simulink model "TParkDir"  (R2020b)
settings: Solver=VariableStepAuto  StartTime=0.0  StopTime=10.0  RelTol=1e-3
values from neighbouring files (symbols this model uses):
  beq = bm+(blnom/(r^2))    (= 1.5e-05)    [valores.m]
  Jeq = (Jm+Jl/r^2)    (= 5.65099476805e-06)    [Valores_de_Parametros.m]    (also in valores.m)
  lambda_m = 0.01546    [Valores_de_Parametros.m]    (also in valores.m)
  Ld = 6.6    [Valores_de_Parametros.m]    (also in valores.m = 0.0066)
  Lls = 0.8    [Valores_de_Parametros.m]    (also in valores.m = 0.0008)
  Lq = 5.8    [Valores_de_Parametros.m]    (also in valores.m = 0.0058)
  Pp = 3    [Valores_de_Parametros.m]    (also in valores.m)
  r = 314.3008    [Valores_de_Parametros.m]    (also in valores.m)
  Rs = 1.02    [Valores_de_Parametros.m]    (also in valores.m)
settings Model: Creator=Matias  LastModifiedBy=Matias

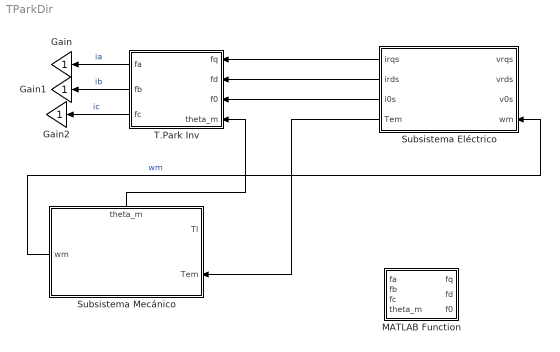
== system TParkDir ==
  Gain : Gain
  Gain1 : Gain
  Gain2 : Gain
  MATLAB Function : MATLAB Function  TreatAsAtomicUnit=on
  Subsistema Eléctrico : Subsystem
  Subsistema Mecánico : Subsystem
      settings: PortSchema="{\"entries\":[{\"content\":{\"sides\":[{\"content\":{\"connectorIds\":[\"In1\",\"In2\"]},\"type\":\"ConnectorPlacement.EquallySpacedRectSide\",\"uuid\":\"ee0e19e9-1195-452b-ab3d-8be3dd040414\"},{\"content\":{\"connectorIds\":[\"Out1\"],\"side\":\"RIGHT\"},\"type\":\"ConnectorPlacement.EquallySpacedRectSide\",\"uuid\":\"524e54e6-4967-4b42-ae12-58774e9397a0\"},{\"content\":{\"connectorIds\":[\"Out2\"],\"side\":\"TOP\"},\"type\":\"ConnectorPlacement.EquallySpacedRectSide\",\"uuid\":\"fab71378-68cb-4446-b02c-df48705d1789\"},{\"content\":{\"connectorIds\":[],\"side\":\"HIDDEN\"},\"type\":\"ConnectorPlacement.EquallySpacedRectSide\",\"uuid\":\"eea92cb8-3517-43ef-96fe-10b46f054d59\"}]},\"type\":\"ConnectorPlacement.EquallySpacedConnector\",\"uuid\":\"156d3ac5-e5c7-4248-8590-4f82c7370a76\"}],\"packageUris\":[\"http://schema.mathworks.com/mf0/Connector/R2020b\"],\"version\":\"1.0\"}"
  T.Park Inv : MATLAB Function  TreatAsAtomicUnit=on
  wires:
  Subsistema Mecánico/1(wm) -> Subsistema Eléctrico/4(wm)  "wm"
  Subsistema Eléctrico/4(Tem) -> Subsistema Mecánico/2(Tem)
  Subsistema Eléctrico/1(irqs) -> T.Park Inv/1(fq)
  Subsistema Eléctrico/2(irds) -> T.Park Inv/2(fd)
  Subsistema Eléctrico/3(i0s) -> T.Park Inv/3(f0)
  Subsistema Mecánico/2(theta_m) -> T.Park Inv/4(theta_m)
  T.Park Inv/1(fa) -> Gain/1  "ia"
  T.Park Inv/2(fb) -> Gain1/1  "ib"
  T.Park Inv/3(fc) -> Gain2/1  "ic"

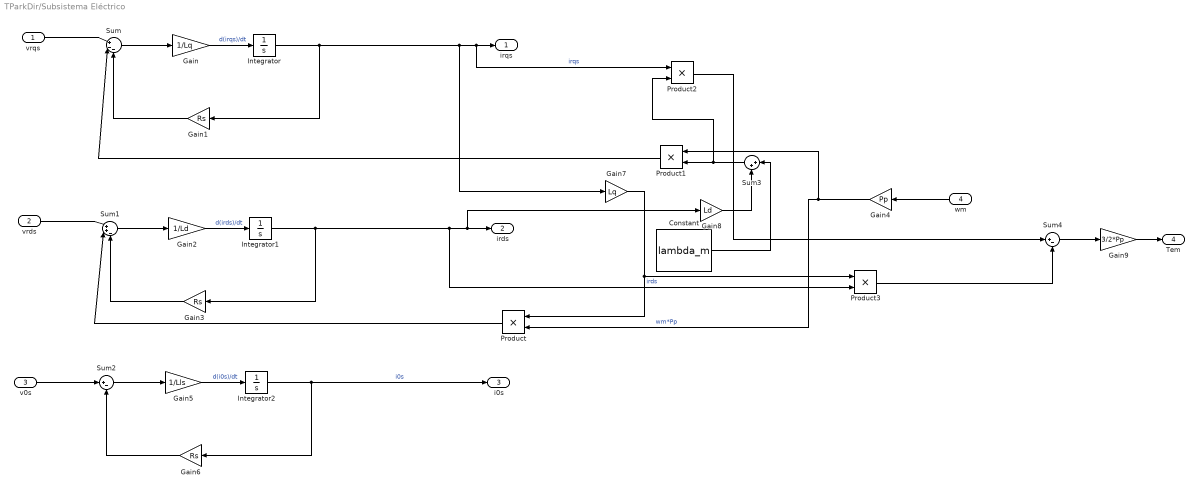
== system TParkDir/Subsistema Eléctrico ==
  vrqs : Inport
  vrds : Inport  Port=2
  v0s : Inport  Port=3
  wm : Inport  Port=4
  Constant : Constant  Value=lambda_m
  Gain : Gain  Gain=1/Lq
  Gain1 : Gain  Gain=Rs
  Gain2 : Gain  Gain=1/Ld
  Gain3 : Gain  Gain=Rs
  Gain4 : Gain  Gain=Pp
  Gain5 : Gain  Gain=1/Lls
  Gain6 : Gain  Gain=Rs
  Gain7 : Gain  Gain=Lq
  Gain8 : Gain  Gain=Ld
  Gain9 : Gain  Gain=3/2*Pp
  Integrator : Integrator
  Integrator1 : Integrator
  Integrator2 : Integrator
  Product{,1..3} (4 alike) : Product
  Sum : Sum  Inputs=|+--
  Sum1 : Sum  Inputs=|++-
  Sum2 : Sum  Inputs=|+-
  Sum3 : Sum  Inputs=|++
  Sum4 : Sum  Inputs=|+-
  irqs : Outport
  irds : Outport  Port=2
  i0s : Outport  Port=3
  Tem : Outport  Port=4
  wires:
  Sum3/1 -> Product2/2, Product1/2
  Integrator1/1 -> Gain3/1, Product3/2, Gain8/1, irds/1  "irds"
  Sum1/1 -> Gain2/1
  Gain8/1 -> Sum3/2
  Gain2/1 -> Integrator1/1  "d(irds)/dt"
  Product2/1 -> Sum4/1
  Constant/1 -> Sum3/1
  Gain3/1 -> Sum1/3
  Sum4/1 -> Gain9/1
  Product3/1 -> Sum4/2
  vrqs/1 -> Sum/1
  wm/1 -> Gain4/1
  vrds/1 -> Sum1/1
  Product/1 -> Sum1/2
  Product1/1 -> Sum/2
  v0s/1 -> Sum2/1
  Gain5/1 -> Integrator2/1  "d(i0s)/dt"
  Sum2/1 -> Gain5/1
  Integrator2/1 -> Gain6/1, i0s/1  "i0s"
  Gain4/1 -> Product1/1, Product/2  "wm*Pp"
  Sum/1 -> Gain/1
  Gain1/1 -> Sum/3
  Gain7/1 -> Product/1, Product3/1
  Integrator/1 -> Gain1/1, Gain7/1, Product2/1, irqs/1  "irqs"
  Gain/1 -> Integrator/1  "d(irqs)/dt"
  Gain9/1 -> Tem/1
  Gain6/1 -> Sum2/2

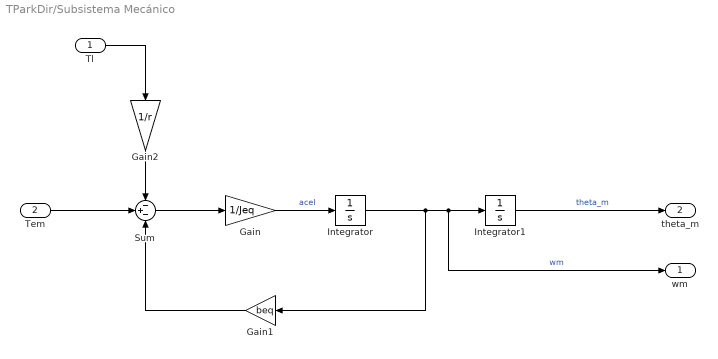
== system TParkDir/Subsistema Mecánico ==
  Tl : Inport
  Tem : Inport  Port=2
  Gain : Gain  Gain=1/Jeq
  Gain1 : Gain  Gain=beq
  Gain2 : Gain  Gain=1/r
  Integrator : Integrator
  Integrator1 : Integrator
  Sum : Sum  Inputs=-+-
  wm : Outport
  theta_m : Outport  Port=2
  wires:
  Sum/1 -> Gain/1
  Tl/1 -> Gain2/1
  Gain1/1 -> Sum/3
  Integrator/1 -> Gain1/1, wm/1, Integrator1/1  "wm"
  Gain2/1 -> Sum/1
  Gain/1 -> Integrator/1  "acel"
  Integrator1/1 -> theta_m/1  "theta_m"
  Tem/1 -> Sum/2

== matlab function TParkDir/MATLAB Function ==
  data: fa input; fq output; fb input; fc input; theta_m input; fd output; f0 output
function [fq,fd,f0] = fcn(fa,fb,fc,theta_m)
fq=2/3*(cos(theta_m)*fa+cos(theta_m-(2*pi/(3)))*fb+cos(theta_m+(2*pi/(3)))*fc);
fd=2/3*(sin(theta_m)*fa+sin(theta_m-(2*pi/(3)))*fb+sin(theta_m+(2*pi/(3)))*fc);
f0=2/3*((1/2)*fa+(1/2)*fb+(1/2)*fc);
y = u;

== matlab function TParkDir/T.Park Inv ==
  data: fq input; fa output; fd input; f0 input; theta_m input; fb output; fc output
function [fa,fb,fc] = fcn(fq,fd,f0,theta_m)
fa=fq*cos(theta_m)+fd*sin(theta_m)+f0;
fb=fq*cos(theta_m-(2*pi/(3)))+fd*sin(theta_m-(2*pi/(3)))+f0;
fc=fq*cos(theta_m+(2*pi/(3)))+fd*sin(theta_m+(2*pi/(3)))+f0;
